simulink model "volumetricEfficiency"  (R2023a)
settings: Solver=VariableStepAuto  StartTime=0.0  StopTime=10.0  RelTol=1e-3
settings Model: Creator=rafael  LastModifiedBy=rafael

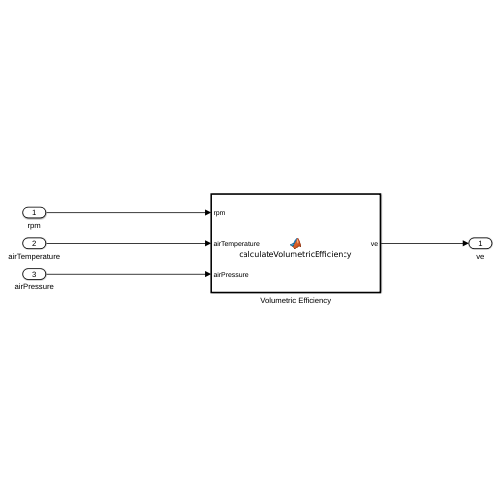
[thumbnail: Simulink's stored preview of the top-level diagram]
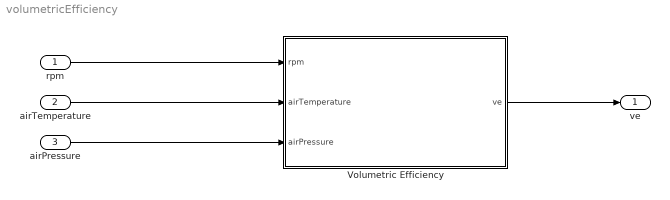
== system volumetricEfficiency ==
  rpm : Inport
  airTemperature : Inport  Port=2
  airPressure : Inport  Port=3
  Volumetric Efficiency : MATLAB Function  Description=Calculate the Volumetric Efficiency considering the current RPM and air pressure and temperature from engine output air flow  TreatAsAtomicUnit=on  RTWFcnName=calculateVolumetricEfficiency  RTWFileName=calculateVolumetricEfficiency
      settings: RTWFileNameOpts=User specified
  ve : Outport
  wires:
  Volumetric Efficiency/1(ve) -> ve/1
  rpm/1 -> Volumetric Efficiency/1(rpm)
  airTemperature/1 -> Volumetric Efficiency/2(airTemperature)
  airPressure/1 -> Volumetric Efficiency/3(airPressure)

== matlab function volumetricEfficiency/Volumetric Efficiency ==
  data: rpm input; ve output; airTemperature input; airPressure input
function ve = calculateVolumetricEfficiency(rpm,airTemperature,airPressure)
    % FUNCTION Calculate Volumetric Efficiency
    %
    % $$ve_{teoric} = V_t \left(\frac{P_{MAP}}{R \cdot T_{MAP}}\right)$$
    % 
    % Args:
    %   rpm: Motor RPM [RPM]
    %   airTemperature: Air Temperature [K]
    %   airPressure: Air Pressure [atm]
    %
    % Returns:
    %   ve: Volumetric Efficiency
    arguments
        rpm (1,1) double {mustBeNumeric,mustBeReal,mustBeNonnegative}
        airTemperature (1,1) double {mustBeNumeric,mustBeReal,mustBePositive}
        airPressure (1,1) double {mustBeNumeric,mustBeReal,mustBePositive}
    end


    % Constants
    R = 8.134;                        % [J/mol*K] Universal Gases Constant
    volumeEngineTotal  = 1.984/1000;  % 1.984 * 10^(-3) [m^3]
    rpmMax = 6000;                    % [RPM] Max RPM Allowed 
    veMax = 1;                        % Max Volumetric Eficiency
    
    veReal = volumeEngineTotal*(airPressure/(R*airTemperature))*(rpm/2)
    veTeoric = volumeEngineTotal*(rpmMax/2)*veMax

    % Full Volumetric Efficience Equation
    % ve = veReal/veTeoric

    % Simplified Volumetric Efficiency Equation
    ve = ((airPressure/(R*airTemperature))*rpm )/(rpmMax*veMax);
end
